simulink model "single_phase_r_circuit"  (R2021b)
settings: Solver=ode23t  StartTime=0.0  StopTime=.2  RelTol=1e-3
libraries: spsSeriesRLCBranchLib x5, spsGroundLib x3, spsVoltageMeasurementLib x2, spsCurrentMeasurementLib x1, spsACVoltageSourceLib x1, spspowerguiLib x1
settings Model: Creator=naeem  LastModifiedBy=tmcnama2
settings SolverCC: AlgebraicLoopSolver=TrustRegion
settings DebuggingCC: SFMachineParentedDataDiag=warning

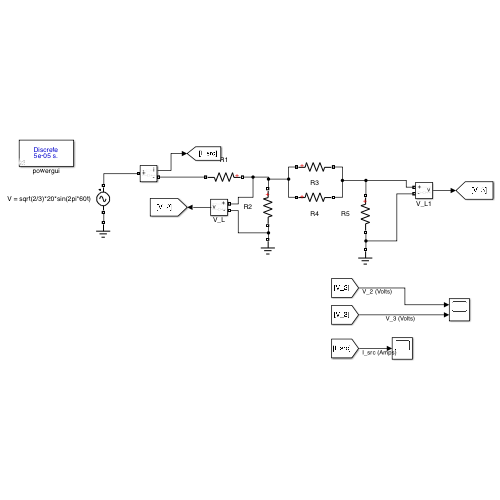
[thumbnail: Simulink's stored preview of the top-level diagram]
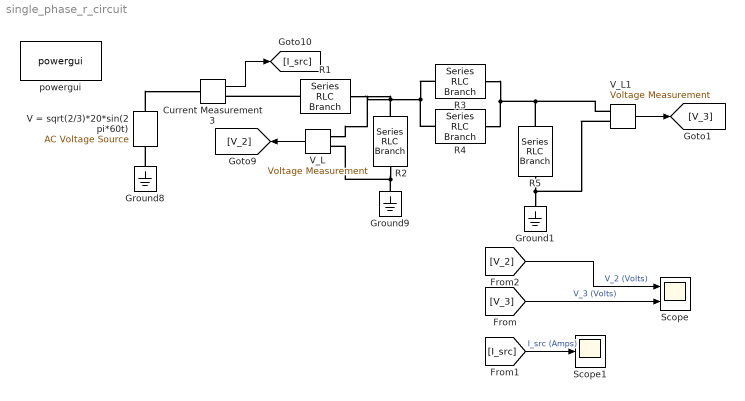
== system single_phase_r_circuit ==
  Current Measurement3 : spsCurrentMeasurementLib/Current Measurement  PhasorSimulation=off  OutputType=Complex  PSBequivalent=0
  Ground1 : spsGroundLib/Ground  LConnTagsString=a
  Ground8 : spsGroundLib/Ground  LConnTagsString=a
  Ground9 : spsGroundLib/Ground  LConnTagsString=a
  R{1..5} (5 alike) : spsSeriesRLCBranchLib/Series RLC Branch  LConnTagsString=__new0  RConnTagsString=__new0  BranchType=R  Resistance=10  Inductance=1e-3  SetiL0=off  InitialCurrent=0  Capacitance=1e-6  Setx0=off  InitialVoltage=0  Measurements=None
  Scope : Scope  NumInputPorts=2
  Scope1 : Scope
  V = sqrt(2/3)*20*sin(2pi*60t) : spsACVoltageSourceLib/AC Voltage Source  Amplitude=20*sqrt(2/3)  Phase=0  Frequency=60  SampleTime=0  Measurements=None  BusType=swing  Pref=10e3  Qref=0  Qmin=-inf  Qmax=+inf
  V_L : spsVoltageMeasurementLib/Voltage Measurement  PhasorSimulation=off  OutputType=Complex  PSBequivalent=0
  V_L1 : spsVoltageMeasurementLib/Voltage Measurement  PhasorSimulation=off  OutputType=Complex  PSBequivalent=0
  powergui : spspowerguiLib/powergui  Priority=1  SimulationMode=Discrete  SampleTime=50e-6  frequency=60  Iterations=50  frequencyindice=60  Pbase=100e6  ErrMax=1e-4  UnitsV=kV  UnitsW=MW  buscounter=0  FunctionMessages=off  echomessages=off  EnableUseOfTLC=off  CurrentSourceSwitches=off  DisableSnubberDevices=off  DisableRonSwitches=off  DisableVfSwitches=off  DisplayEquations=off  AutomaticDiscreteSolvers=off  SolverType=Tustin/Backward Euler (TBE)  Interpol=off  ExternalGateDelay=off  methode=off  Ts=100  x0status=blocks  SPID=on  SwTol=0  HookPort=off  NonlinearTolerance=1e-4  nMaxIteration=100  ContinueOnMaxIteration=off  RestoreLinks=warning  ResistiveCurrentMeasurement=off  Frange=[0:2:500]  Ylog=off  Xlog=on  ShowGrid=off  save=off  variable=ZData  structure=0  ZoomFFT=off  StartTime=0.0  cycles=1  DisplayStyle=1  fundamental=60  FreqAxis=off  MaxFrequency=1000  frequencyindicesteady=1  RmsSteady=1  display=off
  wires:
  V_L/1 -> [V_2]
  Current Measurement3/1 -> [I_src]
  [V_3] -> Scope/2  "V_3 (Volts)"
  V_L1/1 -> [V_3]
  [V_2] -> Scope/1  "V_2 (Volts)"
  [I_src] -> Scope1/1  "I_src (Amps)"
  connections:
  Ground8/LConn1 -- V = sqrt(2/3)*20*sin(2pi*60t)/LConn1
  V = sqrt(2/3)*20*sin(2pi*60t)/RConn1 -- Current Measurement3/LConn1
  R1/RConn1 -- Current Measurement3/RConn1
  R5/RConn1 -- V_L1/LConn2 -- Ground1/LConn1
  R2/LConn1 -- V_L/LConn1 -- R1/LConn1 -- R4/LConn1 -- R3/LConn1
  V_L1/LConn1 -- R5/LConn1 -- R4/RConn1 -- R3/RConn1
  R2/RConn1 -- V_L/LConn2 -- Ground9/LConn1
